simulink model "Problem2"  (R2020a)
settings: Solver=ode23  StartTime=0.0  StopTime=10  RelTol=1e-6  AbsTol=1e-7
PostLoadFcn:
  | sldemo_clutchplot
StartFcn:
  | sldemo_clutchplot Start
StopFcn:
  | if exist ('sldemo_clutch_output')
  |    sldemo_clutchplot Stop
  | end
model workspace (MATLAB code in the model file):
  | % Load initial conditions and other information
  | 
  | load sldemo_clutchparam;
undefined symbols (not defined in the file): be, bv, Ie, Iv, muk, mus, R
CloseFcn:
  | sldemo_clutchplot Close
Description:
  | Building a Clutch Lock-Up Model
  | 
  | This example shows how to use Simulink(R) to model and simulate a
  | rotating clutch system. Although modeling a clutch system is difficult
  | because of topological changes in the system dynamics during lockup, this
  | example shows how Simulinks enabled subsystems feature easily handles
  | such problems. We illustrate how to employ important Simulink modeling
  | concepts in the creation of the clutch simulation. Designers can apply
  | these concepts to many models with strong discontinuities and constraints
  | that may change dynamically.
  | 
  | In the example, we use enabled subsystems to build the clutch
  | model. Two enabled subsystems model the clutch dynamics in either the
  | locked or unlocked position. After running the simulation, a GUI opens.
  | Checking any of the boxes on the GUI produces a plot of any of the
  | selected variables (versus time).
settings Model: ExtModeTrigMode=oneshot  ExtModeArmWhenConnect=off  ExtModeAutoUpdateStatusClock=off  Creator=The MathWorks, Inc.  LastModifiedBy=shweta
settings SolverCC: AutoScaleAbsTol=off
settings DataIOCC: ExternalInput=[]  InitialState=[]  SaveOutput=off  SaveTime=off  ReturnWorkspaceOutputs=off  StateSaveName=x  TimeSaveName=t  OutputSaveName=y  SignalLoggingName=sldemo_clutch_output
settings OptimizationCC: BlockReduction=off  ExpressionDepthLimit=2147483647  InitFltsAndDblsToZero=on  LifeSpan=inf  BufferReusableBoundary=off
settings DebuggingCC: SaveWithParameterizedLinksMsg=none  SignalResolutionControl=TryResolveAllWithWarning  MultiTaskDSMMsg=warning  MultiTaskCondExecSysMsg=none  SigSpecEnsureSampleTimeMsg=none  IntegerOverflowMsg=none  FcnCallInpInsideContextMsg=warning  BusObjectLabelMismatch=none  StateNameClashWarn=warning  SFUnexpectedBacktrackingDiag=warning  SFNoUnconditionalDefaultTransitionDiag=warning  SFExecutionAtInitializationDiag=none  IntegerSaturationMsg=none  ArithmeticOperatorsInVariantConditions=warning
settings HardwareCC: ProdBitPerPointer=32  ProdBitPerSizeT=32  ProdBitPerPtrDiffT=32  ProdLargestAtomicFloat=None  ProdIntDivRoundTo=Undefined  ProdEndianess=Unspecified  ProdWordSize=32  ProdHWDeviceType=32-bit Generic
settings ModelReferenceCC: PropagateSignalLabelsOutOfModel=off
settings SFSimCC: SimUseLocalCustomCode=off  CustomCodeUndefinedFunction=UseInterfaceOnly
settings RTWCC: Description=Generic Real-Time Target  RTWUseLocalCustomCode=off
settings CodeAppCC: StateflowObjectComments=on
settings GRTTargetCC: TargetFcnLib=ansi_tfl_tmw.mat  TargetLangStandard=C89/C90 (ANSI)  CombineOutputUpdateFcns=off  GRTInterface=on
settings ConfigComp: CovMetricSettings=dse  CovSaveCumulativeToWorkspaceVar=on

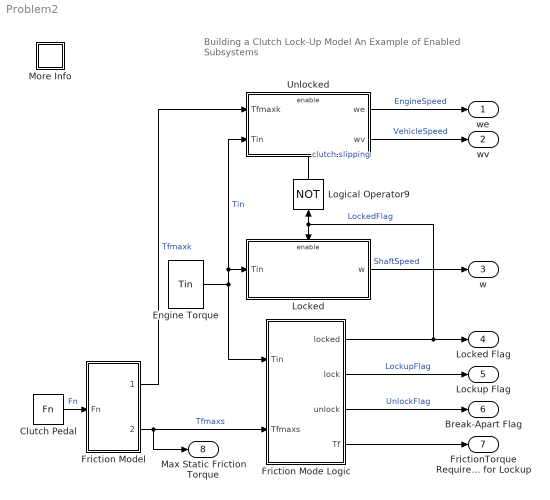
== system Problem2 ==
  note: Building a Clutch Lock-Up Model
      | An Example of Enabled Subsystems
  Clutch Pedal : FromWorkspace  VariableName=Fn  ZeroCross=off
  Engine Torque : FromWorkspace  VariableName=Tin  ZeroCross=off
  Friction Model : Subsystem
  Friction Mode Logic : Subsystem
      mask Display: plot([-3 1 1 3 -1 -1],[-1 -1 1 1 1 -1],-4,-5,4,5)
  Locked : Subsystem  TreatAsAtomicUnit=on
      mask Display: plot(-1,-6,6,12,[0 3],[3 3],[3 1 1 3], [1 1 5 5],[2 4 4 2],[4 4 2 2],[4 5],[3 3])
  Logical Operator9 : Logic  Operator=NOT  Inputs=1  IconShape=distinctive  OutDataTypeStr=boolean
  More Info : Subsystem
      settings: OpenFcn=showExample('simulink_automotive/BuildingAClutchLockUpModelExample')
      mask Display: disp('?')
  Unlocked : Subsystem  TreatAsAtomicUnit=on
      mask Display: plot(-1,-2,6,8,[0 3],[3 3],[3 1 1 3], [1 1 5 5],[2 4 4 2],[4 4 2 2],[4 5],[3 3])
  we : Outport  InitialOutput=0  VectorParamsAs1DForOutWhenUnconnected=off
  wv : Outport  Port=2  InitialOutput=0  VectorParamsAs1DForOutWhenUnconnected=off
  w : Outport  Port=3  InitialOutput=0  VectorParamsAs1DForOutWhenUnconnected=off
  Locked Flag : Outport  Port=4  InitialOutput=0  VectorParamsAs1DForOutWhenUnconnected=off
  Lockup Flag : Outport  Port=5  InitialOutput=0  VectorParamsAs1DForOutWhenUnconnected=off
  Break-Apart Flag : Outport  Port=6  InitialOutput=0  VectorParamsAs1DForOutWhenUnconnected=off
  FrictionTorque Required for Lockup : Outport  Port=7  InitialOutput=0  VectorParamsAs1DForOutWhenUnconnected=off
  Max Static Friction Torque : Outport  Port=8  InitialOutput=0  VectorParamsAs1DForOutWhenUnconnected=off
  wires:
  Friction Mode Logic/3(unlock) -> Break-Apart Flag/1  "UnlockFlag"
  Engine Torque/1 -> Unlocked/2(Tin), Locked/1(Tin), Friction Mode Logic/1(Tin)  "Tin"
  Friction Model/1(Tfmaxk) -> Unlocked/1(Tfmaxk)  "Tfmaxk"
  Unlocked/2(wv) -> wv/1  "VehicleSpeed"
  Unlocked/1(we) -> we/1  "EngineSpeed"
  Friction Mode Logic/1(locked) -> Locked Flag/1, Logical Operator9/1, Locked/Enable  "LockedFlag"
  Friction Mode Logic/2(lock) -> Lockup Flag/1  "LockupFlag"
  Friction Mode Logic/4(Tf) -> FrictionTorque Required for Lockup/1
  Locked/1(w) -> w/1  "ShaftSpeed"
  Logical Operator9/1 -> Unlocked/Enable  "clutch slipping"
  Friction Model/2(Tfmaxs) -> Friction Mode Logic/2(Tfmaxs), Max Static Friction Torque/1  "Tfmaxs"
  Clutch Pedal/1 -> Friction Model/1(Fn)  "Fn"

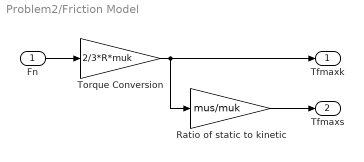
== system Problem2/Friction Model ==
  Fn : Inport
  Ratio of static to kinetic : Gain  Gain=mus/muk  SaturateOnIntegerOverflow=on  OutDataTypeStr=Inherit: Same as input  ParamDataTypeStr=Inherit: Same as input
  Torque Conversion : Gain  Gain=2/3*R*muk  SaturateOnIntegerOverflow=on  OutDataTypeStr=Inherit: Same as input  ParamDataTypeStr=Inherit: Same as input
  Tfmaxk : Outport  InitialOutput=0  VectorParamsAs1DForOutWhenUnconnected=off
  Tfmaxs : Outport  Port=2  InitialOutput=0  VectorParamsAs1DForOutWhenUnconnected=off
  wires:
  Torque Conversion/1 -> Tfmaxk/1, Ratio of static to kinetic/1
  Fn/1 -> Torque Conversion/1
  Ratio of static to kinetic/1 -> Tfmaxs/1

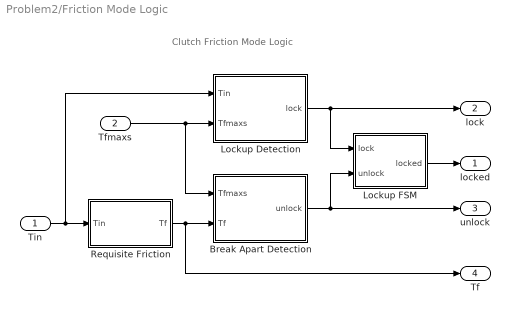
== system Problem2/Friction Mode Logic ==
  note: Clutch Friction Mode Logic
  Tin : Inport
  Tfmaxs : Inport  Port=2
  Break Apart Detection : Subsystem
  Lockup Detection : Subsystem
  Lockup FSM : Subsystem
  Requisite Friction : Subsystem
  locked : Outport  InitialOutput=0  VectorParamsAs1DForOutWhenUnconnected=off
  lock : Outport  Port=2  InitialOutput=0  VectorParamsAs1DForOutWhenUnconnected=off
  unlock : Outport  Port=3  InitialOutput=0  VectorParamsAs1DForOutWhenUnconnected=off
  Tf : Outport  Port=4  InitialOutput=0  VectorParamsAs1DForOutWhenUnconnected=off
  wires:
  Tin/1 -> Lockup Detection/1(Tin), Requisite Friction/1(Tin)
  Tfmaxs/1 -> Lockup Detection/2(Tfmaxs), Break Apart Detection/1(Tfmaxs)
  Requisite Friction/1(Tf) -> Break Apart Detection/2(Tf), Tf/1
  Break Apart Detection/1(unlock) -> Lockup FSM/2(unlock), unlock/1
  Lockup Detection/1(lock) -> Lockup FSM/1(lock), lock/1
  Lockup FSM/1(locked) -> locked/1

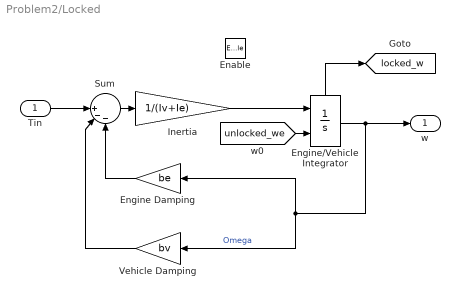
== system Problem2/Locked ==
  Tin : Inport
  Enable : EnablePort  StatesWhenEnabling=reset
  Engine Damping : Gain  Gain=be  SaturateOnIntegerOverflow=on  OutDataTypeStr=Inherit: Same as input  ParamDataTypeStr=Inherit: Same as input
  Engine/Vehicle Integrator : Integrator  InitialConditionSource=external  ShowStatePort=on
  Inertia : Gain  Gain=1/(Iv+Ie)  SaturateOnIntegerOverflow=on  OutDataTypeStr=Inherit: Same as input  ParamDataTypeStr=Inherit: Same as input
  Sum : Sum  Inputs=||+--  InputSameDT=on  SaturateOnIntegerOverflow=on  OutDataTypeStr=Inherit: Same as first input
  Vehicle Damping : Gain  Gain=bv  SaturateOnIntegerOverflow=on  OutDataTypeStr=Inherit: Same as input  ParamDataTypeStr=Inherit: Same as input
  w : Outport  InitialOutput=0  VectorParamsAs1DForOutWhenUnconnected=off
  tag scope: locked_w=global
  wires:
  [unlocked_we] -> Engine/Vehicle Integrator/2
  Engine/Vehicle Integrator/State -> [locked_w]
  Sum/1 -> Inertia/1
  Tin/1 -> Sum/1
  Engine/Vehicle Integrator/1 -> w/1, Engine Damping/1, Vehicle Damping/1  "Omega"
  Engine Damping/1 -> Sum/3
  Inertia/1 -> Engine/Vehicle Integrator/1
  Vehicle Damping/1 -> Sum/2

== system Problem2/More Info ==

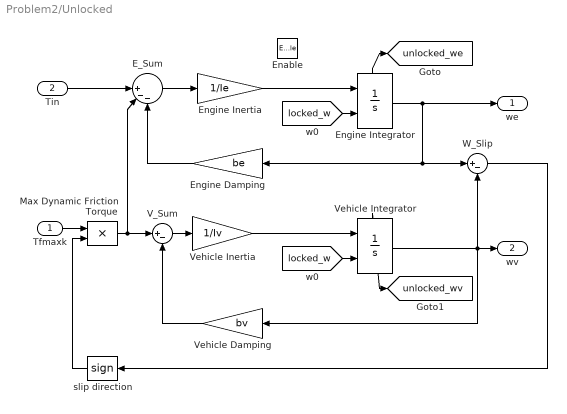
== system Problem2/Unlocked ==
  Tfmaxk : Inport
  Tin : Inport  Port=2
  Enable : EnablePort  StatesWhenEnabling=reset
  E_Sum : Sum  Inputs=||+--  InputSameDT=on  SaturateOnIntegerOverflow=on  OutDataTypeStr=Inherit: Same as first input
  Engine Damping : Gain  Gain=be  SaturateOnIntegerOverflow=on  OutDataTypeStr=Inherit: Same as input  ParamDataTypeStr=Inherit: Same as input
  Engine Inertia : Gain  Gain=1/Ie  SaturateOnIntegerOverflow=on  OutDataTypeStr=Inherit: Same as input  ParamDataTypeStr=Inherit: Same as input
  Engine Integrator : Integrator  InitialConditionSource=external  ShowStatePort=on
  Max Dynamic Friction Torque : Product  InputSameDT=on  RndMeth=Zero  SaturateOnIntegerOverflow=on  OutDataTypeStr=Inherit: Same as first input
  V_Sum : Sum  Inputs=|+-  InputSameDT=on  SaturateOnIntegerOverflow=on  OutDataTypeStr=Inherit: Same as first input
  Vehicle Damping : Gain  Gain=bv  SaturateOnIntegerOverflow=on  OutDataTypeStr=Inherit: Same as input  ParamDataTypeStr=Inherit: Same as input
  Vehicle Inertia : Gain  Gain=1/Iv  SaturateOnIntegerOverflow=on  OutDataTypeStr=Inherit: Same as input  ParamDataTypeStr=Inherit: Same as input
  Vehicle Integrator : Integrator  InitialConditionSource=external  ShowStatePort=on
  W_Slip : Sum  Inputs=|+-  InputSameDT=on  SaturateOnIntegerOverflow=on  OutDataTypeStr=Inherit: Same as first input
  slip direction : Signum
  we : Outport  InitialOutput=0  VectorParamsAs1DForOutWhenUnconnected=off
  wv : Outport  Port=2  InitialOutput=0  VectorParamsAs1DForOutWhenUnconnected=off
  tag scope: unlocked_we=global, unlocked_wv=global
  wires:
  V_Sum/1 -> Vehicle Inertia/1
  Vehicle Damping/1 -> V_Sum/2
  Max Dynamic Friction Torque/1 -> V_Sum/1, E_Sum/2
  Tfmaxk/1 -> Max Dynamic Friction Torque/1
  slip direction/1 -> Max Dynamic Friction Torque/2
  W_Slip/1 -> slip direction/1
  Engine Integrator/State -> [unlocked_we]
  Engine Inertia/1 -> Engine Integrator/1
  E_Sum/1 -> Engine Inertia/1
  Engine Damping/1 -> E_Sum/3
  Engine Integrator/1 -> we/1, Engine Damping/1, W_Slip/1
  [locked_w] -> Engine Integrator/2
  Tin/1 -> E_Sum/1
  Vehicle Integrator/State -> [unlocked_wv]
  [locked_w] -> Vehicle Integrator/2
  Vehicle Inertia/1 -> Vehicle Integrator/1
  Vehicle Integrator/1 -> Vehicle Damping/1, wv/1, W_Slip/2

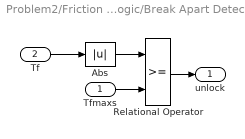
== system Problem2/Friction Mode Logic/Break Apart Detection ==
  Tfmaxs : Inport
  Tf : Inport  Port=2
  Abs : Abs  SaturateOnIntegerOverflow=on
  Relational Operator : RelationalOperator  OutDataTypeStr=boolean  RndMeth=Nearest  InputSameDT=on
  unlock : Outport  InitialOutput=0  VectorParamsAs1DForOutWhenUnconnected=off
  wires:
  Tf/1 -> Abs/1
  Relational Operator/1 -> unlock/1
  Abs/1 -> Relational Operator/1
  Tfmaxs/1 -> Relational Operator/2

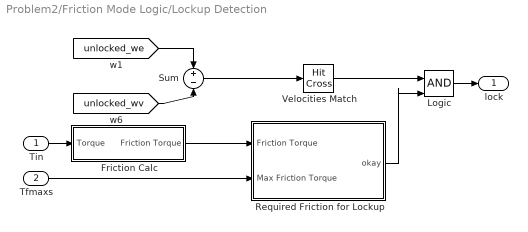
== system Problem2/Friction Mode Logic/Lockup Detection ==
  Tin : Inport
  Tfmaxs : Inport  Port=2
  Friction Calc : Subsystem
  Logic : Logic  IconShape=distinctive  OutDataTypeStr=boolean
  Required Friction for Lockup : Subsystem
  Sum : Sum  Inputs=+-  InputSameDT=on  SaturateOnIntegerOverflow=on  OutDataTypeStr=Inherit: Same as first input
  Velocities Match : HitCross
  lock : Outport  InitialOutput=0  VectorParamsAs1DForOutWhenUnconnected=off
  wires:
  Friction Calc/1(Friction Torque) -> Required Friction for Lockup/1(Friction Torque)
  Tfmaxs/1 -> Required Friction for Lockup/2(Max Friction Torque)
  Velocities Match/1 -> Logic/1
  Logic/1 -> lock/1
  Required Friction for Lockup/1(okay) -> Logic/2
  [unlocked_we] -> Sum/1
  [unlocked_wv] -> Sum/2
  Sum/1 -> Velocities Match/1
  Tin/1 -> Friction Calc/1(Torque)

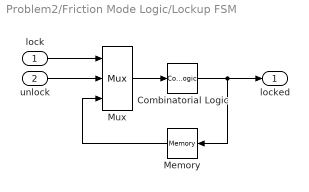
== system Problem2/Friction Mode Logic/Lockup FSM ==
  lock : Inport
  unlock : Inport  Port=2
  Combinatorial Logic : CombinatorialLogic  TruthTable=[0;1;0;0;1;1;1;0]
  Memory : Memory
  Mux : Mux  Inputs=3
  locked : Outport  InitialOutput=0  VectorParamsAs1DForOutWhenUnconnected=off
  wires:
  Memory/1 -> Mux/3
  Combinatorial Logic/1 -> locked/1, Memory/1
  unlock/1 -> Mux/2
  lock/1 -> Mux/1
  Mux/1 -> Combinatorial Logic/1

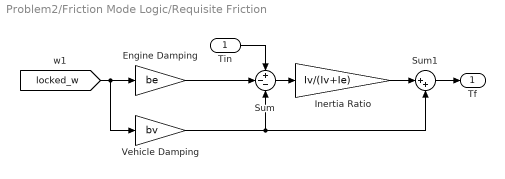
== system Problem2/Friction Mode Logic/Requisite Friction ==
  Tin : Inport
  Engine Damping : Gain  Gain=be  SaturateOnIntegerOverflow=on  OutDataTypeStr=Inherit: Same as input  ParamDataTypeStr=Inherit: Same as input
  Inertia Ratio : Gain  Gain=Iv/(Iv+Ie)  SaturateOnIntegerOverflow=on  OutDataTypeStr=Inherit: Same as input  ParamDataTypeStr=Inherit: Same as input
  Sum : Sum  Inputs=+--  InputSameDT=on  SaturateOnIntegerOverflow=on  OutDataTypeStr=Inherit: Same as first input
  Sum1 : Sum  Inputs=|++  InputSameDT=on  SaturateOnIntegerOverflow=on  OutDataTypeStr=Inherit: Same as first input
  Vehicle Damping : Gain  Gain=bv  SaturateOnIntegerOverflow=on  OutDataTypeStr=Inherit: Same as input  ParamDataTypeStr=Inherit: Same as input
  Tf : Outport  InitialOutput=0  VectorParamsAs1DForOutWhenUnconnected=off
  wires:
  [locked_w] -> Vehicle Damping/1, Engine Damping/1
  Engine Damping/1 -> Sum/2
  Vehicle Damping/1 -> Sum/3, Sum1/2
  Sum/1 -> Inertia Ratio/1
  Tin/1 -> Sum/1
  Inertia Ratio/1 -> Sum1/1
  Sum1/1 -> Tf/1

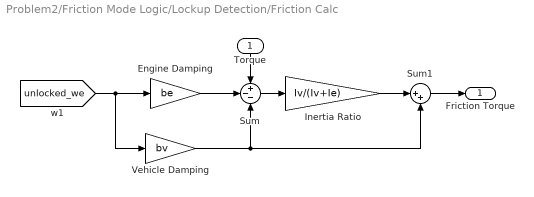
== system Problem2/Friction Mode Logic/Lockup Detection/Friction Calc ==
  Torque : Inport
  Engine Damping : Gain  Gain=be  SaturateOnIntegerOverflow=on  OutDataTypeStr=Inherit: Same as input  ParamDataTypeStr=Inherit: Same as input
  Inertia Ratio : Gain  Gain=Iv/(Iv+Ie)  SaturateOnIntegerOverflow=on  OutDataTypeStr=Inherit: Same as input  ParamDataTypeStr=Inherit: Same as input
  Sum : Sum  Inputs=+--  InputSameDT=on  SaturateOnIntegerOverflow=on  OutDataTypeStr=Inherit: Same as first input
  Sum1 : Sum  Inputs=|++  InputSameDT=on  SaturateOnIntegerOverflow=on  OutDataTypeStr=Inherit: Same as first input
  Vehicle Damping : Gain  Gain=bv  SaturateOnIntegerOverflow=on  OutDataTypeStr=Inherit: Same as input  ParamDataTypeStr=Inherit: Same as input
  Friction Torque : Outport  InitialOutput=0  VectorParamsAs1DForOutWhenUnconnected=off
  wires:
  [unlocked_we] -> Engine Damping/1, Vehicle Damping/1
  Vehicle Damping/1 -> Sum1/2, Sum/3
  Engine Damping/1 -> Sum/2
  Sum/1 -> Inertia Ratio/1
  Torque/1 -> Sum/1
  Inertia Ratio/1 -> Sum1/1
  Sum1/1 -> Friction Torque/1

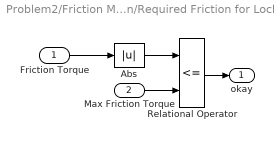
== system Problem2/Friction Mode Logic/Lockup Detection/Required Friction for Lockup ==
  Friction Torque : Inport
  Max Friction Torque : Inport  Port=2
  Abs : Abs  SaturateOnIntegerOverflow=on
  Relational Operator : RelationalOperator  Operator=<=  OutDataTypeStr=boolean  RndMeth=Nearest  InputSameDT=on
  okay : Outport  InitialOutput=0  VectorParamsAs1DForOutWhenUnconnected=off
  wires:
  Friction Torque/1 -> Abs/1
  Relational Operator/1 -> okay/1
  Abs/1 -> Relational Operator/1
  Max Friction Torque/1 -> Relational Operator/2
